simulink model "TorqueFreeMotion"  (R2022b)
settings: Solver=FixedStepAuto  StartTime=0.0  StopTime=tspan  FixedStep=10  RelTol=1e-3
values from neighbouring files (symbols this model uses):
  J = [0.096 0 0; 0 0.096 0; 0 0 0.166]    [ControlledMotionScript.m]    (also in TorqueFreeMotionScript.m = [0.016 0 0; 0 0.016 0; 0 0 0.025])
  T = [0;0;0.31*2]    [TorqueFreeMotionScript.m]
  w_b_0 = [0.000; 0.000; 0.000]    [ControlledMotionScript.m]    (also in TorqueFreeMotionScript.m)
settings Model: Creator=emehiel  LastModifiedBy=bricenrigby
settings SolverCC: AlgebraicLoopSolver=TrustRegion
settings DebuggingCC: UnconnectedInputMsg=warning  UnconnectedOutputMsg=warning  UnconnectedLineMsg=warning  SFMachineParentedDataDiag=warning
settings ModelReferenceCC: EnableRefExpFcnMdlSchedulingChecks=on

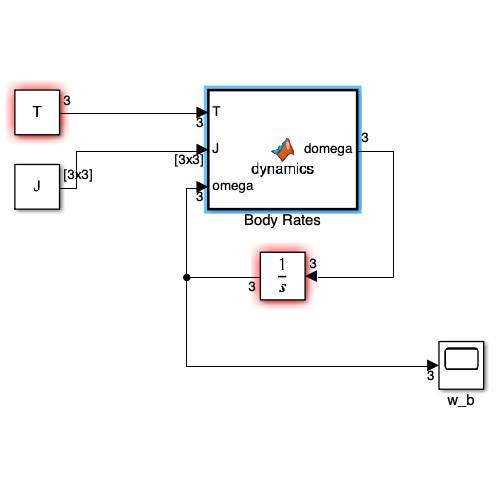
[thumbnail: Simulink's stored preview of the top-level diagram]
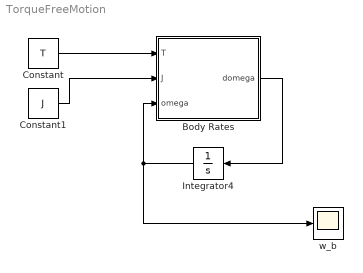
== system TorqueFreeMotion ==
  Body Rates : MATLAB Function  TreatAsAtomicUnit=on
  Constant : Constant  Value=T
  Constant1 : Constant  Value=J
  Integrator4 : Integrator  InitialCondition=w_b_0
  w_b : Scope
  wires:
  Constant/1 -> Body Rates/1(T)
  Constant1/1 -> Body Rates/2(J)
  Body Rates/1(domega) -> Integrator4/1
  Integrator4/1 -> Body Rates/3(omega), w_b/1

== matlab function TorqueFreeMotion/Body Rates ==
  data: T input; J input; omega input; domega output
function domega = dynamics(T, J, omega)
%#codegen

% Compute the derivative of the angular velocity $\omega$ here
Ix = J(1,1);
Iy = J(2,2);
Iz = J(3,3);

T1 = T(1);
T2 = T(2);
T3 = T(3);

wdot1 = (T1 - (Iz-Iy)*omega(2)*omega(3))/Ix;
wdot2 = (T2 - (Ix-Iz)*omega(1)*omega(3))/Iy;
wdot3 = (T3 - (Iy-Ix)*omega(1)*omega(2))/Iz;

domega = [wdot1; wdot2; wdot3];
end
